simulink model "statefeedback_1"  (R2022b)
settings: Solver=VariableStepAuto  StartTime=0.0  StopTime=10  RelTol=1e-3
values from neighbouring files (symbols this model uses):
  A = parameters{1}    [state_feedback.m]
  B = parameters{2}    [state_feedback.m]
  C = parameters{3}    [state_feedback.m]
  K_calculated = K_ba*T    [state_feedback.m]
  x0 = parameters{5}    [state_feedback.m]
settings Model: Creator=wyton  LastModifiedBy=wanrylin
settings SolverCC: AlgebraicLoopSolver=TrustRegion
settings DataIOCC: SaveState=on
settings DebuggingCC: UnconnectedInputMsg=warning  UnconnectedOutputMsg=warning  UnconnectedLineMsg=warning  SFMachineParentedDataDiag=warning
settings ModelReferenceCC: EnableRefExpFcnMdlSchedulingChecks=on
settings RTWCC: DLArmComputeVersion=19.05

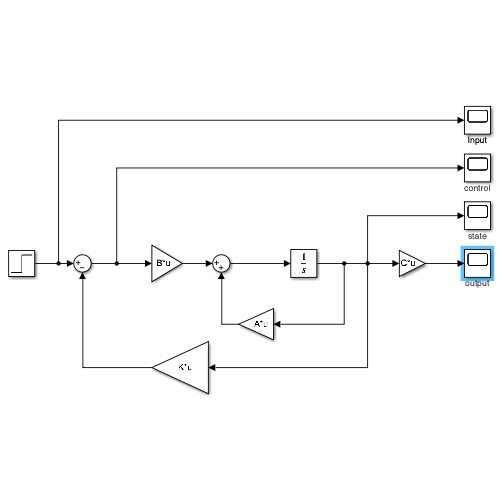
[thumbnail: Simulink's stored preview of the top-level diagram]
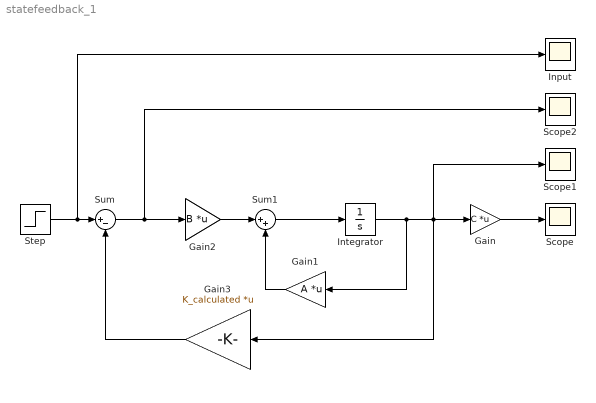
== system statefeedback_1 ==
  Gain : Gain  Gain=C  Multiplication=Matrix(K*u)
  Gain1 : Gain  Gain=A  Multiplication=Matrix(K*u)
  Gain2 : Gain  Tag=B  Gain=B  Multiplication=Matrix(K*u)
  Gain3 : Gain  Gain=K_calculated  Multiplication=Matrix(K*u)
  Input : Scope
  Integrator : Integrator  InitialCondition=x0
  Scope : Scope
      settings: AttributesFormatString=output
  Scope1 : Scope
      settings: AttributesFormatString=state
  Scope2 : Scope
      settings: AttributesFormatString=control
  Step : Step  Time=0  Before=[0,0]  After=[0,0]  SampleTime=0
  Sum : Sum  Inputs=|+-
  Sum1 : Sum  Inputs=|++
  wires:
  Step/1 -> Input/1, Sum/1
  Sum/1 -> Scope2/1, Gain2/1
  Sum1/1 -> Integrator/1
  Gain2/1 -> Sum1/1
  Integrator/1 -> Gain1/1, Gain3/1, Gain/1, Scope1/1
  Gain1/1 -> Sum1/2
  Gain/1 -> Scope/1
  Gain3/1 -> Sum/2
